simulink model "sterowanie"  (R2022b)
settings: Solver=VariableStepAuto  StartTime=0.0  StopTime=tmax  MaxStep=2  RelTol=1e-3
values from neighbouring files (symbols this model uses):
  dTwew = 1    [obliczenia.m]
  k1 = (20.2553 - 20)/0.0100000000000000    (= 25.53)    [obliczenia.m]    (also in obliczenia2.m = 65.8)
  k2 = (20.2553 - 20)/0.0100000000000000    (= 25.53)    [obliczenia.m]
  Ki = 1    [obliczenia.m]    (also in obliczenia2.m = 0)
  Kp = 0.9*Tczas1/(k1*Topu1)    (= 0.199057468577)    [obliczenia.m]    (also in obliczenia2.m = 1.05226274907)
  Tczas1 = 25390-Topu1    (= 21570)    [obliczenia.m]    (also in obliczenia2.m = 12463)
  Tczas2 = 21425-11955    (= 9470)    [obliczenia.m]
  Ti = 3.33*Topu1/Kp    (= 63904.1583866)    [obliczenia.m]    (also in obliczenia2.m = 11755.1763626)
  Topu1 = 5820- 2000    (= 3820)    [obliczenia.m]    (also in obliczenia2.m = 1080)
  Topu2 = 21425 - Tczas2    (= 11955)    [obliczenia.m]
  tsok = 2000    [obliczenia.m]    (also in obliczenia2.m = 80000)
  Twew10 = (Cpw*Fmg10 *Kcg*Tgz10 + Kcw*(Kcg + Cpw*Fmg10)*Tzew0)/(Kcg*Kcw + Cpw*Fmg10*(Kcg + Kcw))    (= 20)    [obliczenia.m]    (also in obliczenia2.m)
libraries: slpidlib x2
settings Model: Creator=asialalala  LastModifiedBy=asialalala
settings DataIOCC: ReturnWorkspaceOutputs=off

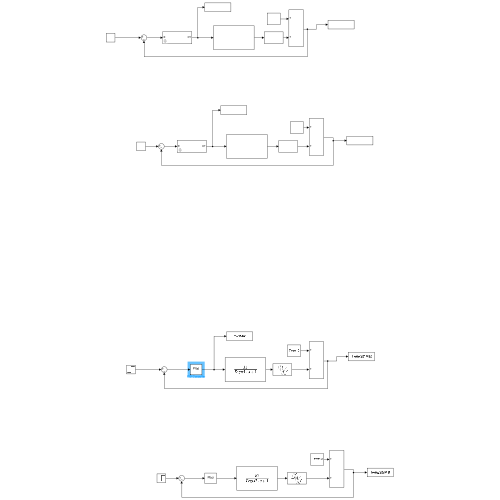
[thumbnail: Simulink's stored preview of the top-level diagram]
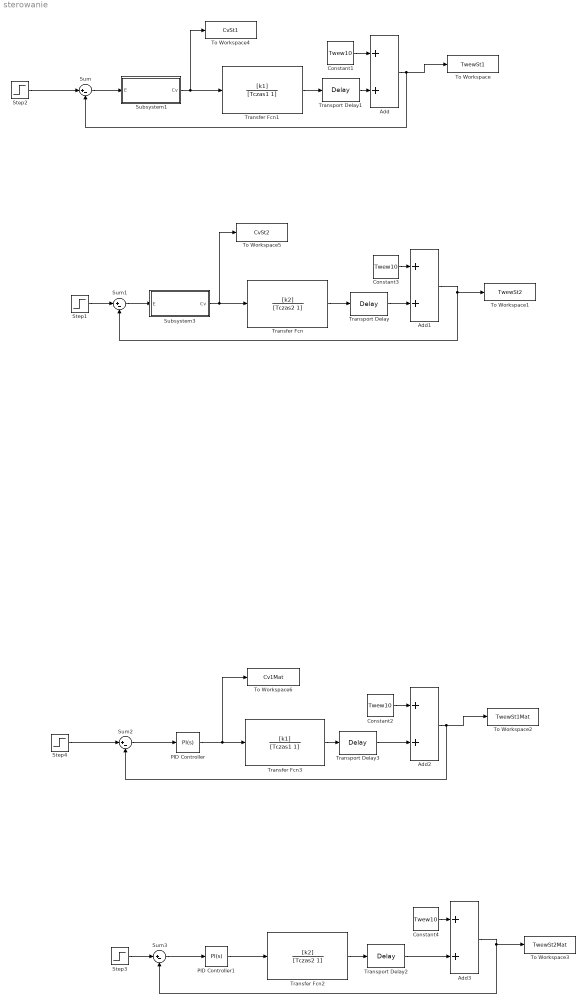
== system sterowanie ==
  Add{,1..3} (4 alike) : Sum
  Constant{1..4} (4 alike) : Constant  Value=Twew10
  PID Controller : slpidlib/PID Controller  Controller=PI  Form=Parallel  TimeDomain=Continuous-time  UseExternalTs=off  SampleTime=-1  IntegratorMethod=Forward Euler  FilterMethod=Forward Euler  ControllerParametersSource=internal  P=0.06016  I=4.35489929311168e-06  UseKiTs=off  D=0  N=100  UseFilter=on  TunerSelectOption=Transfer Function Based (PID Tuner App)  InitialConditionSource=internal  InitialConditionForIntegrator=0  InitialConditionForFilter=0  DifferentiatorICPrevScaledInput=0  ExternalReset=none  TrackingMode=off  Kt=1  LimitOutput=off  SatLimitsSource=internal  UpperSaturationLimit=inf  LowerSaturationLimit=-inf  LinearizeAsGain=on  AntiWindupMode=none  Kb=1  LimitIntegrator=off  UpperIntegratorSaturationLimit=inf  LowerIntegratorSaturationLimit=-inf  POutMin=[]  POutMax=[]  IOutMin=[]  IOutMax=[]  DOutMin=[]  DOutMax=[]  NOutMin=[]  NOutMax=[]  SumOutMin=[]  SumOutMax=[]  SaturationOutMin=[]  SaturationOutMax=[]  PParamMin=[]  PParamMax=[]  IParamMin=[]  IParamMax=[]  DParamMin=[]  DParamMax=[]  NParamMin=[]  NParamMax=[]  KbParamMin=[]  KbParamMax=[]  KtParamMin=[]  KtParamMax=[]  KbOutMin=[]  KbOutMax=[]  KtOutMin=[]  KtOutMax=[]  IntegratorOutMin=[]  IntegratorOutMax=[]  FilterOutMin=[]  FilterOutMax=[]  SumI1OutMin=[]  SumI1OutMax=[]  SumI2OutMin=[]  SumI2OutMax=[]  SumI3OutMin=[]  SumI3OutMax=[]  SumI4OutMin=[]  SumI4OutMax=[]  SumDOutMin=[]  SumDOutMax=[]  DifferentiatorOutMin=[]  DifferentiatorOutMax=[]  FilterDiffOutCoefMin=[]  FilterDiffOutCoefMax=[]  ReciprocalOutMin=[]  ReciprocalOutMax=[]  SumDenOutMin=[]  SumDenOutMax=[]  SumNumOutMin=[]  SumNumOutMax=[]  DivideOutMin=[]  DivideOutMax=[]  UdiffTsProdOutMin=[]  UdiffTsProdOutMax=[]  NTsProdOutMin=[]  NTsProdOutMax=[]  UintegralTsProdOutMin=[]  UintegralTsProdOutMax=[]  UngainTsProdOutMin=[]  UngainTsProdOutMax=[]  ClampingZeroOutDataTypeStr=Inherit: Inherit via back propagation  ClampingZeroOutMin=[]  ClampingZeroOutMax=[]  FilterDenConstantOutDataTypeStr=Inherit: Inherit via back propagation  FilterDenConstantOutMin=[]  FilterDenConstantOutMax=[]  PCopyOutDataTypeStr=Inherit: Inherit via back propagation  PCopyOutMin=[]  PCopyOutMax=[]  NCopyOutDataTypeStr=Inherit: Inherit via back propagation  NCopyOutMin=[]  NCopyOutMax=[]  IntegratorContinuousStateAttributes=''  IntegratorStateMustResolveToSignalObject=off  IntegratorRTWStateStorageClass=Auto  FilterContinuousStateAttributes=''  FilterStateMustResolveToSignalObject=off  FilterRTWStateStorageClass=Auto  ParallelPVariant=InternalParameters  IdealPVariant=Disabled  IVariant=InternalParameters  DVariant=Disabled  IntegratorVariant=Continuous  SatVariant=Disabled  AWVariant=Passthrough  PCopyVariant=Disabled  TRVariant=Disabled  FdbkBlocksVariant=Forward  IdealPFdbkVariant=Disabled  SatFdbkVariant=Disabled  DerivativeFilterVariant=Disabled  NVariant=Disabled  NCopyVariant=Disabled_SignalSpec  FilterICVariant=Disabled  IntegratorICVariant=InternalICs  ExternalResetVariant=Disabled  TRSumVariant=Passthrough  SumFdbkVariant=Disabled  SumVariant=Sum_PI  TsampFilterVariant=InternalTs  TsampNgainVariant=Passthrough  TsampIntegralVariant=Passthrough  ExternalSaturationOutDataTypeStr=Inherit: Same as second input
  PID Controller1 : slpidlib/PID Controller  Controller=PI  Form=Parallel  TimeDomain=Continuous-time  UseExternalTs=off  SampleTime=-1  IntegratorMethod=Forward Euler  FilterMethod=Forward Euler  ControllerParametersSource=internal  P=Kp  I=1/Ti  UseKiTs=off  D=0  N=100  UseFilter=on  TunerSelectOption=Transfer Function Based (PID Tuner App)  InitialConditionSource=internal  InitialConditionForIntegrator=0  InitialConditionForFilter=0  DifferentiatorICPrevScaledInput=0  ExternalReset=none  TrackingMode=off  Kt=1  LimitOutput=off  SatLimitsSource=internal  UpperSaturationLimit=inf  LowerSaturationLimit=-inf  LinearizeAsGain=on  AntiWindupMode=none  Kb=1  LimitIntegrator=off  UpperIntegratorSaturationLimit=inf  LowerIntegratorSaturationLimit=-inf  POutMin=[]  POutMax=[]  IOutMin=[]  IOutMax=[]  DOutMin=[]  DOutMax=[]  NOutMin=[]  NOutMax=[]  SumOutMin=[]  SumOutMax=[]  SaturationOutMin=[]  SaturationOutMax=[]  PParamMin=[]  PParamMax=[]  IParamMin=[]  IParamMax=[]  DParamMin=[]  DParamMax=[]  NParamMin=[]  NParamMax=[]  KbParamMin=[]  KbParamMax=[]  KtParamMin=[]  KtParamMax=[]  KbOutMin=[]  KbOutMax=[]  KtOutMin=[]  KtOutMax=[]  IntegratorOutMin=[]  IntegratorOutMax=[]  FilterOutMin=[]  FilterOutMax=[]  SumI1OutMin=[]  SumI1OutMax=[]  SumI2OutMin=[]  SumI2OutMax=[]  SumI3OutMin=[]  SumI3OutMax=[]  SumI4OutMin=[]  SumI4OutMax=[]  SumDOutMin=[]  SumDOutMax=[]  DifferentiatorOutMin=[]  DifferentiatorOutMax=[]  FilterDiffOutCoefMin=[]  FilterDiffOutCoefMax=[]  ReciprocalOutMin=[]  ReciprocalOutMax=[]  SumDenOutMin=[]  SumDenOutMax=[]  SumNumOutMin=[]  SumNumOutMax=[]  DivideOutMin=[]  DivideOutMax=[]  UdiffTsProdOutMin=[]  UdiffTsProdOutMax=[]  NTsProdOutMin=[]  NTsProdOutMax=[]  UintegralTsProdOutMin=[]  UintegralTsProdOutMax=[]  UngainTsProdOutMin=[]  UngainTsProdOutMax=[]  ClampingZeroOutDataTypeStr=Inherit: Inherit via back propagation  ClampingZeroOutMin=[]  ClampingZeroOutMax=[]  FilterDenConstantOutDataTypeStr=Inherit: Inherit via back propagation  FilterDenConstantOutMin=[]  FilterDenConstantOutMax=[]  PCopyOutDataTypeStr=Inherit: Inherit via back propagation  PCopyOutMin=[]  PCopyOutMax=[]  NCopyOutDataTypeStr=Inherit: Inherit via back propagation  NCopyOutMin=[]  NCopyOutMax=[]  IntegratorContinuousStateAttributes=''  IntegratorStateMustResolveToSignalObject=off  IntegratorRTWStateStorageClass=Auto  FilterContinuousStateAttributes=''  FilterStateMustResolveToSignalObject=off  FilterRTWStateStorageClass=Auto  ParallelPVariant=InternalParameters  IdealPVariant=Disabled  IVariant=InternalParameters  DVariant=Disabled  IntegratorVariant=Continuous  SatVariant=Disabled  AWVariant=Passthrough  PCopyVariant=Disabled  TRVariant=Disabled  FdbkBlocksVariant=Forward  IdealPFdbkVariant=Disabled  SatFdbkVariant=Disabled  DerivativeFilterVariant=Disabled  NVariant=Disabled  NCopyVariant=Disabled_SignalSpec  FilterICVariant=Disabled  IntegratorICVariant=InternalICs  ExternalResetVariant=Disabled  TRSumVariant=Passthrough  SumFdbkVariant=Disabled  SumVariant=Sum_PI  TsampFilterVariant=InternalTs  TsampNgainVariant=Passthrough  TsampIntegralVariant=Passthrough  ExternalSaturationOutDataTypeStr=Inherit: Same as second input
  Step{1..4} (4 alike) : Step  Time=tsok  Before=Twew10  After=dTwew + Twew10  SampleTime=0
  Subsystem1 : Subsystem  mask{Kp=Kp, Ti=Ti, Cv0=0, Ki=Ki}
  Subsystem3 : Subsystem  mask{Kp=Kp, Ti=Ti, Cv0=0, Ki=Ki}
  Sum{,1..3} (4 alike) : Sum  Inputs=|+-
  To Workspace : ToWorkspace  VariableName=TwewSt1  SampleTime=-1
  To Workspace1 : ToWorkspace  VariableName=TwewSt2  SampleTime=-1
  To Workspace2 : ToWorkspace  VariableName=TwewSt1Mat  SampleTime=-1
  To Workspace3 : ToWorkspace  VariableName=TwewSt2Mat  SampleTime=-1
  To Workspace4 : ToWorkspace  VariableName=CvSt1  SampleTime=-1
  To Workspace5 : ToWorkspace  VariableName=CvSt2  SampleTime=-1
  To Workspace6 : ToWorkspace  VariableName=Cv1Mat  SampleTime=-1
  Transfer Fcn : TransferFcn  Numerator=[k2]  Denominator=[Tczas2 1]
  Transfer Fcn1 : TransferFcn  Numerator=[k1]  Denominator=[Tczas1 1]
  Transfer Fcn2 : TransferFcn  Numerator=[k2]  Denominator=[Tczas2 1]
  Transfer Fcn3 : TransferFcn  Numerator=[k1]  Denominator=[Tczas1 1]
  Transport Delay : TransportDelay  DelayTime=Topu2
  Transport Delay1 : TransportDelay  DelayTime=Topu1
  Transport Delay2 : TransportDelay  DelayTime=Topu2
  Transport Delay3 : TransportDelay  DelayTime=Topu1
  wires:
  Add/1 -> Sum/2, To Workspace/1
  Constant1/1 -> Add/1
  Sum1/1 -> Subsystem3/1(E)
  Add1/1 -> Sum1/2, To Workspace1/1
  Constant3/1 -> Add1/1
  Step2/1 -> Sum/1
  Subsystem1/1(Cv) -> To Workspace4/1, Transfer Fcn1/1
  Subsystem3/1(Cv) -> To Workspace5/1, Transfer Fcn/1
  Transfer Fcn/1 -> Transport Delay/1
  Transport Delay/1 -> Add1/2
  Transfer Fcn1/1 -> Transport Delay1/1
  Transport Delay1/1 -> Add/2
  Sum/1 -> Subsystem1/1(E)
  Step1/1 -> Sum1/1
  Transport Delay3/1 -> Add2/2
  Add2/1 -> Sum2/2, To Workspace2/1
  Constant2/1 -> Add2/1
  Sum3/1 -> PID Controller1/1
  Transfer Fcn2/1 -> Transport Delay2/1
  PID Controller/1 -> To Workspace6/1, Transfer Fcn3/1
  Constant4/1 -> Add3/1
  Step3/1 -> Sum3/1
  Step4/1 -> Sum2/1
  Add3/1 -> Sum3/2, To Workspace3/1
  PID Controller1/1 -> Transfer Fcn2/1
  Transport Delay2/1 -> Add3/2
  Sum2/1 -> PID Controller/1
  Transfer Fcn3/1 -> Transport Delay3/1

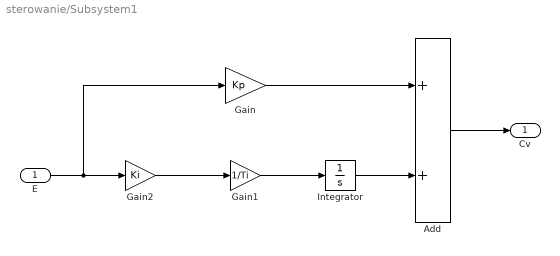
== system sterowanie/Subsystem1 ==
  E : Inport
  Add : Sum
  Gain : Gain  Gain=Kp
  Gain1 : Gain  Gain=1/Ti
  Gain2 : Gain  Gain=Ki
  Integrator : Integrator  InitialCondition=Cv0
  Cv : Outport
  wires:
  E/1 -> Gain/1, Gain2/1
  Gain2/1 -> Gain1/1
  Gain1/1 -> Integrator/1
  Add/1 -> Cv/1
  Gain/1 -> Add/1
  Integrator/1 -> Add/2

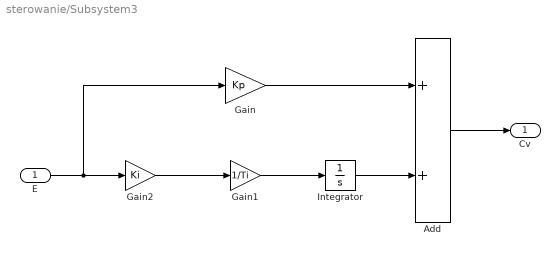
== system sterowanie/Subsystem3 ==
  E : Inport
  Add : Sum
  Gain : Gain  Gain=Kp
  Gain1 : Gain  Gain=1/Ti
  Gain2 : Gain  Gain=Ki
  Integrator : Integrator  InitialCondition=Cv0
  Cv : Outport
  wires:
  E/1 -> Gain/1, Gain2/1
  Gain2/1 -> Gain1/1
  Gain1/1 -> Integrator/1
  Add/1 -> Cv/1
  Gain/1 -> Add/1
  Integrator/1 -> Add/2
